simulink model "MatlabNonlinearStateEstimationForActuatorDelay"  (R2020b)
settings: Solver=VariableStepAuto  StartTime=0.0  StopTime=10  RelTol=1e-3
PostLoadFcn:
  | t0 = 0;
values from neighbouring files (symbols this model uses):
  cg = temp(4)    [NonlinearStateEstimationForActuatorDelay.m]
  Croll = Croll_p + .0001 * (rand - 0.5)    [Forces_and_Moments_Calculator.m]
  Cside = 0    [Forces_and_Moments_Calculator.m]
  Cyaw = Cyaw + .1 * (rand - 0.5)    [Forces_and_Moments_Calculator.m]
  F = eye(6)    [MEKFAttitudeOnly.m]
  I = reshape(x(1:9), [3 3])    [AdaptiveLQR.m]    (also in MEKF.m = diag([0.08 0.08 0.002]); MEKFAttitudeOnly.m = diag([0.08 0.08 0.002]); MEKF_old.m = diag([0.08 0.08 0.002]); NonlinearStateEstimationForActuatorDelay.m = diag([Ixx, Ixx, Izz]))
  mass = 1.0565    [ImpactVelocityNotParallelMatlab.m]    (also in NonlinearStateEstimationForActuatorDelay.m = temp(1); OneDLanding.m; RunImpactVelocityParforCompiled.m; Tracker.m = 1.0616753546)
  q = x(13:16)    [AdaptiveLQR.m]    (also in MEKF.m = nominal_state(4:7); MEKFAttitudeOnly.m = [1 0 0 0]; MEKF_old.m = nominal_state(4:7); NonlinearStateEstimationForActuatorDelay.m = x(4:7))
  r = sym('r', [3 1])    [StateSpaceController.m]    (also in TimeDelayCompensationElevator.m = [0;0]; Tracker.m = [0; 0; -(rocket_length - Average_cg)])
  ThrustTable = xlsread('F15_Thrust','Sheet1')    [ImpactVelocityNotParallelMatlab.m]    (also in OneDLanding.m; ParallelImpactVelocity.m; RunImpactVelocityParforCompiled.m)
undefined symbols (not defined in the file or in its folder): Earth, HeightAboveSeaLevel, Light, masscgI, MIL, WGS84
libraries: shared6dof x5, simulink x3, aerolibwind2 x3, vrlib x2, sharedutil x2, aerolibasang x2, shared6dofsys x2, sharedtransform x2, aerolibatmos2 x1, aerolibbdyn x1, aerolibconvert2 x1, aerolibtransform2 x1
(part 1 of 2)
settings Model: SimulationMode=accelerator  Creator=rag  LastModifiedBy=rag
settings OptimizationCC: InitFltsAndDblsToZero=on
settings HardwareCC: ProdLongLongMode=on  TargetLongLongMode=on

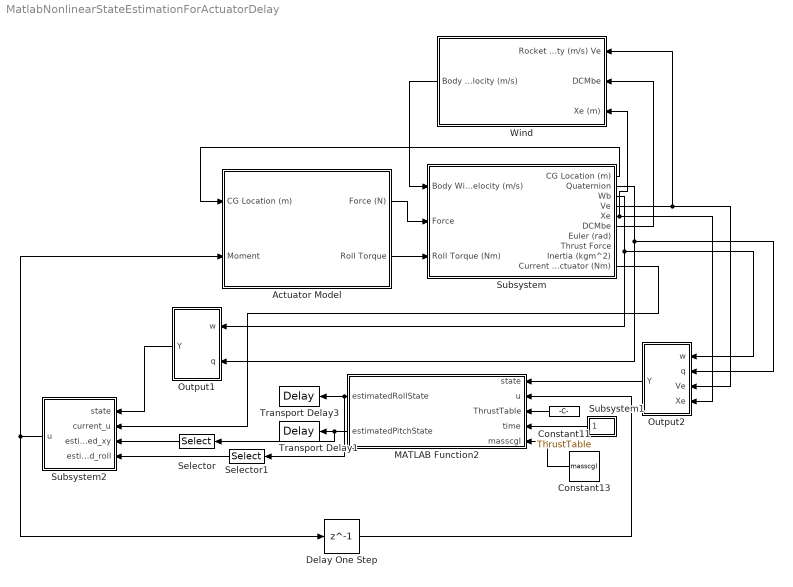
== system MatlabNonlinearStateEstimationForActuatorDelay ==
  Actuator Model : Subsystem
  Constant11 : Constant  Value=ThrustTable
  Constant13 : Constant  Value=masscgI
  Delay One Step : Delay  DelayLength=1
  MATLAB Function2 : MATLAB Function  TreatAsAtomicUnit=on  SystemSampleTime=0.001
  Output1 : Subsystem
  Output2 : Subsystem
  Selector : Selector  InputPortWidth=15  IndexOptions=Index vector (dialog)  Indices=[1:9]  OutputSizes=1
  Selector1 : Selector  InputPortWidth=15  IndexOptions=Index vector (dialog)  Indices=[1:9]  OutputSizes=1
  Subsystem : Subsystem
  Subsystem1 : Subsystem
  Subsystem2 : Subsystem
  Transport Delay1 : TransportDelay  DelayTime=.07  TransDelayFeedthrough=on
  Transport Delay3 : TransportDelay  DelayTime=.01  TransDelayFeedthrough=on
  Wind : Subsystem
  wires:
  Actuator Model/2(Roll Torque) -> Subsystem/3(Roll Torque (Nm))
  Actuator Model/1(Force (N)) -> Subsystem/2(Force)
  Subsystem/1(CG Location (m)) -> Actuator Model/1(CG Location (m))
  Output2/1(Y) -> MATLAB Function2/1(state)
  Subsystem/3(Wb) -> Output2/1(w), Output1/1(w)
  Subsystem/2(Quaternion) -> Output2/2(" q"), Output1/2(" q")
  Subsystem/4(Ve) -> Wind/1(Rocket velocity (m/s) Ve), Output2/3(Ve)
  Subsystem/5(Xe) -> Wind/3(Xe (m)), Output2/4(Xe)
  Subsystem2/1(u) -> Actuator Model/2(Moment), Delay One Step/1
  Constant11/1 -> MATLAB Function2/3(ThrustTable)
  Subsystem1/1(time) -> MATLAB Function2/4(time)
  Constant13/1 -> MATLAB Function2/5(masscgI)
  Output1/1(Y) -> Subsystem2/1(state)
  MATLAB Function2/1(estimatedRollState) -> Transport Delay3/1, Selector1/1
  MATLAB Function2/2(estimatedPitchState) -> Selector/1, Transport Delay1/1
  Delay One Step/1 -> MATLAB Function2/2(u)
  Selector/1 -> Subsystem2/3(estimated_xy)
  Selector1/1 -> Subsystem2/4(estimated_roll)
  Subsystem/10(Current Actuator (Nm)) -> Subsystem2/2(current_u)
  Wind/1(Body Wind Velocity (m/s)) -> Subsystem/1(Body Wind Velocity (m/s))
  Subsystem/6(DCMbe) -> Wind/2(DCMbe)

== system MatlabNonlinearStateEstimationForActuatorDelay/Actuator Model ==
  CG Location (m) : Inport
  Moment : Inport  Port=2
  Constant14 : Constant  Value=[0 1; -1 0]
  Constant3 : Constant  Value=.95
  Demux2 : Demux  Outputs=3
  Force : Product  Multiplication=Matrix(*)
  Moment to Force : Product  Inputs=/*
  Mux2 : Mux  Inputs=2
  Rate Transition : RateTransition  OutPortSampleTime=0.02
  Sum1 : Sum  Inputs=-+|
  Transport Delay : TransportDelay  DelayTime=0.07  TransDelayFeedthrough=on
  Transport Delay1 : TransportDelay  DelayTime=0.01  TransDelayFeedthrough=on
  Force (N) : Outport
  Roll Torque : Outport  Port=2
  wires:
  Demux2/1 -> Mux2/1
  Mux2/1 -> Transport Delay/1
  Sum1/1 -> Moment to Force/1
  Moment to Force/1 -> Force/2
  Constant3/1 -> Sum1/2
  Demux2/2 -> Mux2/2
  Moment/1 -> Demux2/1
  Constant14/1 -> Force/1
  Demux2/3 -> Transport Delay1/1
  CG Location (m)/1 -> Sum1/1
  Force/1 -> Force (N)/1
  Transport Delay/1 -> Moment to Force/2
  Transport Delay1/1 -> Roll Torque/1

== system MatlabNonlinearStateEstimationForActuatorDelay/Output1 ==
  w : Inport
  " q" : Inport  Port=2
  Integrator1 : Integrator
  Selector1 : Selector  InputPortWidth=4  IndexOptions=Index vector (dialog)  Indices=[2 3 4]  OutputSizes=1
  Vector Concatenate4 : Concatenate  NumInputs=3
  Y : Outport  VectorParamsAs1DForOutWhenUnconnected=off
  wires:
  Vector Concatenate4/1 -> Y/1
  w/1 -> Vector Concatenate4/1
  " q"/1 -> Selector1/1
  Integrator1/1 -> Vector Concatenate4/3
  Selector1/1 -> Vector Concatenate4/2, Integrator1/1

== system MatlabNonlinearStateEstimationForActuatorDelay/Output2 ==
  w : Inport
  " q" : Inport  Port=2
  Ve : Inport  Port=3
  Xe : Inport  Port=4
  Integrator1 : Integrator
  Selector1 : Selector  InputPortWidth=4  IndexOptions=Index vector (dialog)  Indices=[2 3 4]  OutputSizes=1
  Vector Concatenate4 : Concatenate  NumInputs=5
  Y : Outport  VectorParamsAs1DForOutWhenUnconnected=off
  wires:
  Vector Concatenate4/1 -> Y/1
  w/1 -> Vector Concatenate4/1
  " q"/1 -> Selector1/1, Vector Concatenate4/2
  Integrator1/1 -> Vector Concatenate4/3
  Selector1/1 -> Integrator1/1
  Xe/1 -> Vector Concatenate4/5
  Ve/1 -> Vector Concatenate4/4

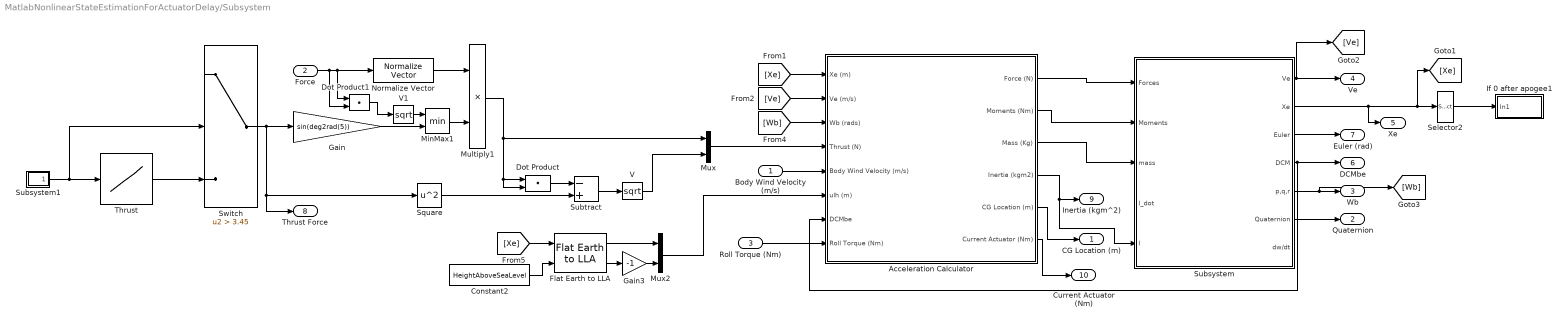
== system MatlabNonlinearStateEstimationForActuatorDelay/Subsystem ==
  Body Wind Velocity (m/s) : Inport
  Force : Inport  Port=2  PortDimensions=2
  Roll Torque (Nm) : Inport  Port=3
  Acceleration Calculator : Subsystem
  Constant2 : Constant  Value=HeightAboveSeaLevel
  Dot Product : DotProduct  SaturateOnIntegerOverflow=on  OutDataTypeStr=Inherit: Inherit via internal rule
  Dot Product1 : DotProduct  SaturateOnIntegerOverflow=on  OutDataTypeStr=Inherit: Inherit via internal rule
  Flat Earth to LLA : aerolibtransform2/Flat Earth to LLA  units=Metric (MKS)  ptype=Earth (WGS84)  F=1/298.257223563  R=6378137  refPosPort=off  LL0=[21.318358277648 -157.9232805920725]  psi=0
  Gain : Gain  Gain=sin(deg2rad(5))
  Gain3 : Gain  Gain=-1
  If 0 after apogee1 : Subsystem
  MinMax1 : MinMax  Inputs=2
  Multiply1 : Product  Inputs=**
  Mux : Mux  Inputs=2
  Mux2 : Mux  Inputs=2
  Normalize Vector : vrlib/Utilities/Normalize Vector  maxzero=0
  Selector2 : Selector  InputPortWidth=3  IndexOptions=Index vector (dialog)  Indices=[3]  OutputSizes=1
  Square : Math  Operator=square  SignedPower=on  SaturateOnIntegerOverflow=on
  Subsystem : Subsystem
  Subsystem1 : Subsystem
  Subtract : Sum  Inputs=-+
  Switch : Switch  Criteria=u2 > Threshold  Threshold=3.45
  Thrust : Lookup_n-D  NumberOfTableDimensions=1  BreakpointsForDimension1=ThrustTable(:,1)  BreakpointsForDimension1FirstPoint=0  BreakpointsForDimension1Spacing=1.5e-5  Table=ThrustTable(:,2)  ExtrapMethod=Clip  InternalRulePriority=Speed  RndMeth=Simplest  InputSameDT=on
  V : Math  Operator=sqrt  SignedPower=on  SaturateOnIntegerOverflow=on
  V1 : Math  Operator=sqrt  SignedPower=on  SaturateOnIntegerOverflow=on
  CG Location (m) : Outport  VectorParamsAs1DForOutWhenUnconnected=off
  Quaternion : Outport  Port=2  VectorParamsAs1DForOutWhenUnconnected=off
  Wb : Outport  Port=3  VectorParamsAs1DForOutWhenUnconnected=off
  Ve : Outport  Port=4  VectorParamsAs1DForOutWhenUnconnected=off
  Xe : Outport  Port=5  VectorParamsAs1DForOutWhenUnconnected=off
  DCMbe : Outport  Port=6  VectorParamsAs1DForOutWhenUnconnected=off
  Euler (rad) : Outport  Port=7  VectorParamsAs1DForOutWhenUnconnected=off
  Thrust Force : Outport  Port=8  VectorParamsAs1DForOutWhenUnconnected=off
  Inertia (kgm^2) : Outport  Port=9  VectorParamsAs1DForOutWhenUnconnected=off
  Current Actuator (Nm) : Outport  Port=10
  wires:
  Flat Earth to LLA/1 -> Mux2/1
  Flat Earth to LLA/2 -> Gain3/1
  Gain3/1 -> Mux2/2
  Mux2/1 -> Acceleration Calculator/6(ulh (m))
  Constant2/1 -> Flat Earth to LLA/2
  [Xe] -> Acceleration Calculator/1(Xe (m))
  Selector2/1 -> If 0 after apogee1/1(In1)
  [Xe] -> Flat Earth to LLA/1
  Acceleration Calculator/5(CG Location (m)) -> CG Location (m)/1
  Acceleration Calculator/4(Inertia (kgm2)) -> Subsystem/5(I), Inertia (kgm^2)/1
  Acceleration Calculator/1(Force (N)) -> Subsystem/1(Forces)
  Roll Torque (Nm)/1 -> Acceleration Calculator/8(Roll Torque (Nm))
  Gain/1 -> MinMax1/2
  Switch/1 -> Thrust Force/1, Square/1, Gain/1
  Subsystem1/1(time) -> Switch/2, Thrust/1
  Subsystem/2(Xe) -> Xe/1, [Xe], Selector2/1
  Subsystem/3(Euler) -> Euler (rad)/1
  Square/1 -> Subtract/2
  Dot Product/1 -> Subtract/1
  V/1 -> Mux/2
  Subtract/1 -> V/1
  Dot Product1/1 -> V1/1
  MinMax1/1 -> Multiply1/2
  Normalize Vector/1 -> Multiply1/1
  V1/1 -> MinMax1/1
  Force/1 -> Dot Product1/2, Dot Product1/1, Normalize Vector/1
  Subsystem/6(Quaternion) -> Quaternion/1
  Subsystem/4(DCM) -> Acceleration Calculator/7(DCMbe), DCMbe/1
  Thrust/1 -> Switch/3
  Acceleration Calculator/2(Moments (Nm)) -> Subsystem/2(Moments)
  Multiply1/1 -> Mux/1, Dot Product/2, Dot Product/1
  Body Wind Velocity (m/s)/1 -> Acceleration Calculator/5(Body Wind Velocity (m/s))
  Acceleration Calculator/3(Mass (Kg)) -> Subsystem/3(mass)
  Subsystem/1(Ve) -> [Ve], Ve/1
  [Ve] -> Acceleration Calculator/2(Ve (m/s))
  Mux/1 -> Acceleration Calculator/4(Thrust (N))
  Subsystem/5(p,q,r) -> [Wb], Wb/1
  [Wb] -> Acceleration Calculator/3(Wb (rads))
  Acceleration Calculator/6(Current Actuator (Nm)) -> Current Actuator (Nm)/1

== system MatlabNonlinearStateEstimationForActuatorDelay/Subsystem1 ==
  Clock : Clock
      settings: Decimation=100
  Constant : Constant  Value=t0
  Sum : Sum  Inputs=|++
  time : Outport
  wires:
  Clock/1 -> Sum/1
  Sum/1 -> time/1
  Constant/1 -> Sum/2

== system MatlabNonlinearStateEstimationForActuatorDelay/Subsystem2 ==
  state : Inport
  current_u : Inport  Port=2
  estimated_xy : Inport  Port=3
  estimated_roll : Inport  Port=4
  Clock : Clock
  MATLAB Function1 : MATLAB Function  TreatAsAtomicUnit=on
  Matrix Multiply : Product  Multiplication=Matrix(*)
  Matrix Multiply1 : Product  Multiplication=Matrix(*)
  Mux : Mux  Inputs=2
  Sum : Sum  Inputs=|--
  u : Outport
  wires:
  Clock/1 -> MATLAB Function1/2(time)
  state/1 -> MATLAB Function1/1(state)
  Sum/1 -> u/1
  MATLAB Function1/3(k_0_out) -> Sum/2
  MATLAB Function1/1(K_x_xy_out) -> Matrix Multiply/1
  current_u/1 -> MATLAB Function1/3(current_u)
  MATLAB Function1/2(K_x_roll_out) -> Matrix Multiply1/1
  estimated_xy/1 -> Matrix Multiply/2
  estimated_roll/1 -> Matrix Multiply1/2
  Matrix Multiply/1 -> Mux/1
  Matrix Multiply1/1 -> Mux/2
  Mux/1 -> Sum/1

== system MatlabNonlinearStateEstimationForActuatorDelay/Wind ==
  Rocket velocity (m/s) Ve : Inport
  DCMbe : Inport  Port=2
  Xe (m) : Inport  Port=3
  Constant : Constant  Commented=on  Value=2
  Ground : Ground  Commented=on
  Mux : Mux  Commented=on  Inputs=3
  Sel2 : Selector  InputPortWidth=3  IndexOptions=Index vector (dialog)  Indices=3  OutputSizes=1
  Subsystem3 : Subsystem
  Terminator : Terminator
  transform to body axes : shared6dof/6DOF (Euler Angles)/transform to Inertial axes   Commented=on  SystemSampleTime=-1  VariantActivationTime=update diagram  Latency=0  AutoFrameSizeCalculation=off
      settings: SourceProductBaseCode=AE,PW,MT,UV,VE,VP
  Body Wind Velocity (m/s) : Outport  VectorParamsAs1DForOutWhenUnconnected=off
  wires:
  DCMbe/1 -> Subsystem3/3(DCMbe), transform to body axes/2
  Rocket velocity (m/s) Ve/1 -> Subsystem3/1(Rocket velocity (m/s) Ve)
  Mux/1 -> transform to body axes/1
  Xe (m)/1 -> Sel2/1
  Constant/1 -> Mux/1
  Subsystem3/1(wind angular velocity (rad/s)) -> Terminator/1
  Sel2/1 -> Subsystem3/2(height (m))
  Ground/1 -> Mux/2, Mux/3
  Subsystem3/2(body axis wind velocity (m/s)) -> Body Wind Velocity (m/s)/1

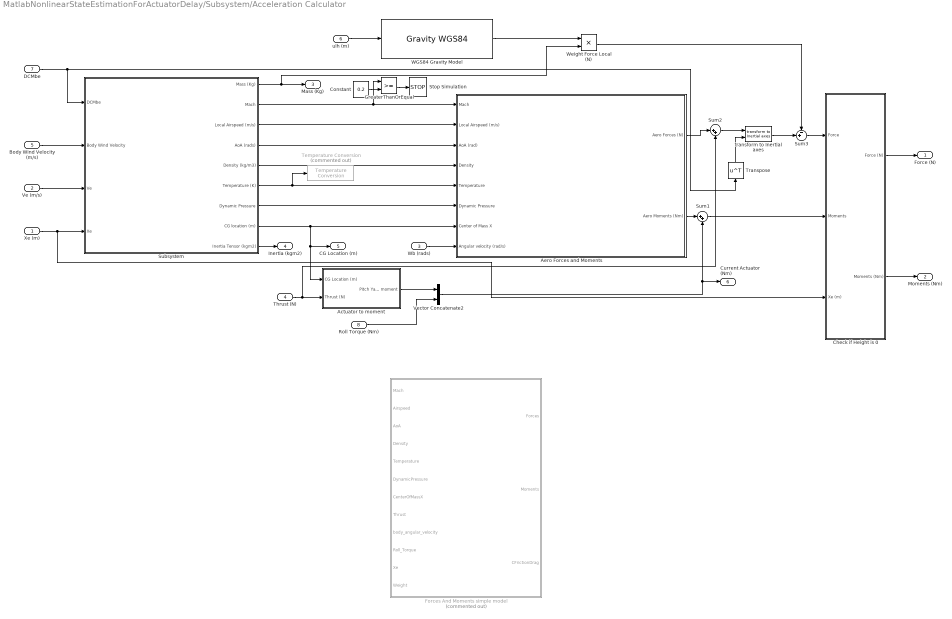
== system MatlabNonlinearStateEstimationForActuatorDelay/Subsystem/Acceleration Calculator ==
  Xe (m) : Inport
  Ve (m/s) : Inport  Port=2
  Wb (rads) : Inport  Port=3
  Thrust (N) : Inport  Port=4
  Body Wind Velocity (m/s) : Inport  Port=5
  ulh (m) : Inport  Port=6  PortDimensions=3
  DCMbe : Inport  Port=7
  Roll Torque (Nm) : Inport  Port=8
  Actuator to moment : Subsystem
  Aero Forces and Moments : Subsystem
  Check if Height is 0 : Subsystem
  Constant : Constant  Value=0.2
  Forces And Moments simple model : MATLAB Function  Commented=on  TreatAsAtomicUnit=on
  GreaterThanOrEqual : RelationalOperator  OutDataTypeStr=boolean  RndMeth=Simplest
  Stop Simulation : Stop
  Subsystem : Subsystem
  Sum1 : Sum  Inputs=|++
  Sum2 : Sum  Inputs=|++
  Sum3 : Sum  Inputs=-+|
  Temperature Conversion : aerolibconvert2/Temperature Conversion  Commented=on  IU=K  OU=C
      settings: SourceProductBaseCode=AE
  Transpose : Math  Operator=transpose  SignedPower=on  SaturateOnIntegerOverflow=on
  Vector Concatenate2 : Concatenate
  "WGS84 Gravity Model  " : GravityWGS84
  Weight Force Local (N) : Product
  "transform to Inertial axes " : shared6dof/6DOF (Euler Angles)/transform to Inertial axes   SystemSampleTime=-1  VariantActivationTime=update diagram  Latency=0  AutoFrameSizeCalculation=off
      settings: SourceProductBaseCode=AE,PW,MT,UV,VE,VP
  Force (N) : Outport  VectorParamsAs1DForOutWhenUnconnected=off
  Moments (Nm) : Outport  Port=2  VectorParamsAs1DForOutWhenUnconnected=off
  Mass (Kg) : Outport  Port=3  VectorParamsAs1DForOutWhenUnconnected=off
  Inertia (kgm2) : Outport  Port=4  VectorParamsAs1DForOutWhenUnconnected=off
  CG Location (m) : Outport  Port=5  VectorParamsAs1DForOutWhenUnconnected=off
  Current Actuator (Nm) : Outport  Port=6
  wires:
  Ve (m/s)/1 -> Subsystem/3(Ve)
  Subsystem/9(Inertia Tensor (kgm2)) -> Inertia (kgm2)/1
  Subsystem/1(Mass (Kg)) -> Weight Force Local (N)/2, Mass (Kg)/1
  DCMbe/1 -> Transpose/1, Subsystem/1(DCMbe)
  ulh (m)/1 -> "WGS84 Gravity Model  "/1
  Roll Torque (Nm)/1 -> Vector Concatenate2/2
  Thrust (N)/1 -> Sum2/2, Actuator to moment/2(Thrust (N))
  Actuator to moment/1(Pitch Yaw moment) -> Vector Concatenate2/1
  Xe (m)/1 -> Subsystem/4(Xe), Check if Height is 0/3(Xe (m))
  Subsystem/3(Local Airspeed (m/s)) -> Aero Forces and Moments/2(Local Airspeed (m/s))
  Subsystem/2(Mach) -> GreaterThanOrEqual/1, Aero Forces and Moments/1(Mach)
  Subsystem/4(AoA (rads)) -> Aero Forces and Moments/3(AoA (rad))
  Subsystem/5(Density (kg/m3)) -> Aero Forces and Moments/4(Density)
  Subsystem/6(Temperature (K)) -> Temperature Conversion/1, Aero Forces and Moments/5(Temperature)
  Subsystem/7(Dynamic Pressure) -> Aero Forces and Moments/6(Dynamic Pressure)
  Subsystem/8(CG location (m)) -> Aero Forces and Moments/7(Center of Mass X), Actuator to moment/1(CG Location (m)), CG Location (m)/1
  Wb (rads)/1 -> Aero Forces and Moments/8(Angular velocity (rad/s))
  Aero Forces and Moments/1(Aero Forces (N)) -> Sum2/1
  Weight Force Local (N)/1 -> Sum3/1
  Sum1/1 -> Check if Height is 0/2(Moments)
  Sum2/1 -> "transform to Inertial axes "/1
  Check if Height is 0/1(Force (N)) -> Force (N)/1
  Check if Height is 0/2(Moments (Nm)) -> Moments (Nm)/1
  Body Wind Velocity (m/s)/1 -> Subsystem/2(Body Wind Velocity)
  "WGS84 Gravity Model  "/1 -> Weight Force Local (N)/1
  Constant/1 -> GreaterThanOrEqual/2
  GreaterThanOrEqual/1 -> Stop Simulation/1
  Transpose/1 -> "transform to Inertial axes "/2
  "transform to Inertial axes "/1 -> Sum3/2
  Sum3/1 -> Check if Height is 0/1(Force)
  Aero Forces and Moments/2(Aero Moments (Nm)) -> Sum1/1
  Vector Concatenate2/1 -> Current Actuator (Nm)/1, Sum1/2

== system MatlabNonlinearStateEstimationForActuatorDelay/Subsystem/If 0 after apogee1 ==
  In1 : Inport
  Compare To Zero1 : simulink/Logic and Bit Operations/Compare To Zero  relop=<=  OutDataTypeStr=boolean
  Constant3 : Constant  Value=0.5
  Logical Operator1 : Logic  AllPortsSameDT=off  OutDataTypeStr=boolean
  Relational Operator1 : RelationalOperator  Operator=>  OutDataTypeStr=boolean  RndMeth=Simplest
  Stop Simulation1 : Stop
  Subsystem1 : Subsystem
  wires:
  Constant3/1 -> Relational Operator1/2
  In1/1 -> Compare To Zero1/1
  Logical Operator1/1 -> Stop Simulation1/1
  Compare To Zero1/1 -> Logical Operator1/2
  Relational Operator1/1 -> Logical Operator1/1
  Subsystem1/1(time) -> Relational Operator1/1

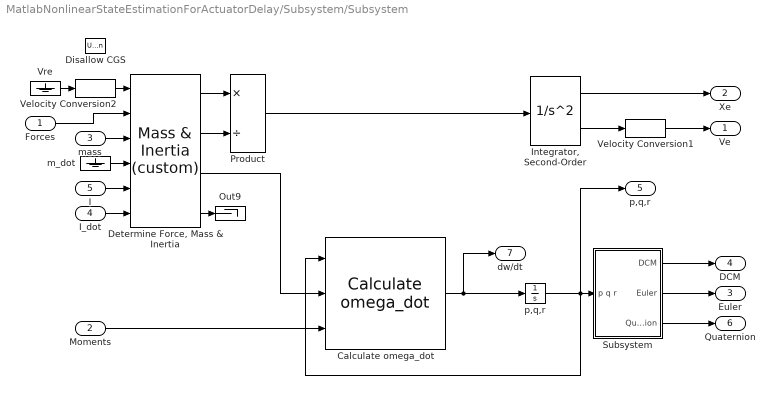
== system MatlabNonlinearStateEstimationForActuatorDelay/Subsystem/Subsystem ==
  Forces : Inport  Unit=N  PortDimensions=3
  Moments : Inport  Port=2  Unit=N*m  PortDimensions=3
  mass : Inport  Port=3  Unit=kg
  I_dot : Inport  Port=4  Unit=kg*m^2/s  PortDimensions=[3 3]
  I : Inport  Port=5  Unit=kg*m^2  PortDimensions=[3 3]
  Calculate omega_dot : shared6dofsys/Calculate omega_dot  aMode=aMode
      settings: SourceProductBaseCode=AE,PW,MT,UV,VE,VP
  "Determine Force, Mass & Inertia" : shared6dofsys/Mass & Inertia (custom)  aMode=aMode
      settings: SourceProductBaseCode=AE,PW,MT,UV,VE,VP
  Disallow CGS : UnitConfiguration  UnitSystemsStr=English,SI,SI (extended)  AllowAllUnitSystems=off
  "Integrator, Second-Order" : SecondOrderIntegrator  ICX=[0 0 50]  LimitX=on  LowerLimitX=[-inf -inf 0]  ICDXDT=0
  Out9 : Terminator
  Product : Product  Inputs=*/  SaturateOnIntegerOverflow=on  OutDataTypeStr=Inherit: Same as first input
  Subsystem : Subsystem
  Velocity Conversion1 : shared6dof/6DOF (Euler Angles)/Velocity Conversion1  SystemSampleTime=-1  VariantActivationTime=update diagram  Latency=0  AutoFrameSizeCalculation=off
      settings: SourceProductBaseCode=AE,PW,MT,UV,VE,VP
  Velocity Conversion2 : shared6dof/6DOF (Euler Angles)/Velocity Conversion2  SystemSampleTime=-1  VariantActivationTime=update diagram  Latency=0  AutoFrameSizeCalculation=off
      settings: SourceProductBaseCode=AE,PW,MT,UV,VE,VP
  Vre : Ground
  m_dot : Ground
  "p,q,r " : Integrator  InitialCondition=[0 0 0]
  Ve : Outport  Unit=m/s  VectorParamsAs1DForOutWhenUnconnected=off
  Xe : Outport  Port=2  Unit=m  VectorParamsAs1DForOutWhenUnconnected=off
  Euler : Outport  Port=3  Unit=rad  VectorParamsAs1DForOutWhenUnconnected=off
  DCM : Outport  Port=4  Unit=1  VectorParamsAs1DForOutWhenUnconnected=off
  p,q,r : Outport  Port=5  Unit=rad/s  VectorParamsAs1DForOutWhenUnconnected=off
  Quaternion : Outport  Port=6  VectorParamsAs1DForOutWhenUnconnected=off
  dw/dt : Outport  Port=7  VectorParamsAs1DForOutWhenUnconnected=off
  wires:
  Subsystem/2(Euler) -> Euler/1
  "Determine Force, Mass & Inertia"/3 -> Calculate omega_dot/2
  "p,q,r "/1 -> Subsystem/1(p q r), p,q,r/1, Calculate omega_dot/1
  Product/1 -> "Integrator, Second-Order"/1
  mass/1 -> "Determine Force, Mass & Inertia"/3
  Velocity Conversion1/1 -> Ve/1
  Subsystem/1(DCM) -> DCM/1
  Calculate omega_dot/1 -> dw/dt/1, "p,q,r "/1
  Forces/1 -> "Determine Force, Mass & Inertia"/2
  "Determine Force, Mass & Inertia"/4 -> Out9/1
  I_dot/1 -> "Determine Force, Mass & Inertia"/6
  I/1 -> "Determine Force, Mass & Inertia"/5
  Velocity Conversion2/1 -> "Determine Force, Mass & Inertia"/1
  Vre/1 -> Velocity Conversion2/1
  "Determine Force, Mass & Inertia"/1 -> Product/1
  "Determine Force, Mass & Inertia"/2 -> Product/2
  m_dot/1 -> "Determine Force, Mass & Inertia"/4
  Subsystem/3(Quaternion) -> Quaternion/1
  "Integrator, Second-Order"/2 -> Velocity Conversion1/1
  "Integrator, Second-Order"/1 -> Xe/1
  Moments/1 -> Calculate omega_dot/3

== system MatlabNonlinearStateEstimationForActuatorDelay/Subsystem/Subsystem1 ==
  Clock : Clock
      settings: Decimation=100
  Constant : Constant  Value=t0
  Sum : Sum  Inputs=|++
  time : Outport
  wires:
  Clock/1 -> Sum/1
  Sum/1 -> time/1
  Constant/1 -> Sum/2

== system MatlabNonlinearStateEstimationForActuatorDelay/Wind/Subsystem3 ==
  Rocket velocity (m/s) Ve : Inport
  height (m) : Inport  Port=2
  DCMbe : Inport  Port=3
  Discrete Wind Gust Model : aerolibwind2/Discrete Wind Gust Model  units=Metric (MKS)  Gx=on  Gy=on  Gz=on  t_0=GustStart  d_m=GustLength  v_m=GuestAmplitude
  Dot Product : DotProduct  SaturateOnIntegerOverflow=on  OutDataTypeStr=Inherit: Inherit via internal rule
  Sum : Sum  Inputs=3
  V : Math  Operator=sqrt  SignedPower=on  SaturateOnIntegerOverflow=on
  Von Karman Wind Turbulence Model (Continuous (+q +r)) : aerolibwind2/Dryden Wind Turbulence Model  (Continuous (+q -r))  units=Metric (MKS)  spec=MIL-F-8785C  model=Discrete Dryden (+q -r)  W20=ShearSpeed  Wdeg=ShearDirection  TurbProb=10^-2 - Light  L_high=762  Wingspan=1  ts=0.1  Seed=[23341 23342 23343 23344]  T_on=on
  Wind Shear Model : aerolibwind2/Wind Shear Model  units=Metric (MKS)  phase=Category C - Terminal Flight Phase  W_20=ShearSpeed  Wdeg=ShearDirection
  wind angular velocity (rad/s) : Outport  VectorParamsAs1DForOutWhenUnconnected=off
  body axis wind velocity (m/s) : Outport  Port=2  VectorParamsAs1DForOutWhenUnconnected=off
  wires:
  height (m)/1 -> Wind Shear Model/1, Von Karman Wind Turbulence Model (Continuous (+q +r))/1
  Discrete Wind Gust Model/1 -> Sum/1
  DCMbe/1 -> Wind Shear Model/2, Von Karman Wind Turbulence Model (Continuous (+q +r))/3
  V/1 -> Von Karman Wind Turbulence Model (Continuous (+q +r))/2, Discrete Wind Gust Model/1
  Sum/1 -> body axis wind velocity (m/s)/1
  Wind Shear Model/1 -> Sum/3
  Von Karman Wind Turbulence Model (Continuous (+q +r))/1 -> Sum/2
  Von Karman Wind Turbulence Model (Continuous (+q +r))/2 -> wind angular velocity (rad/s)/1
  Dot Product/1 -> V/1
  Rocket velocity (m/s) Ve/1 -> Dot Product/1, Dot Product/2

== system MatlabNonlinearStateEstimationForActuatorDelay/Subsystem/Acceleration Calculator/Actuator to moment ==
  CG Location (m) : Inport
  Thrust (N) : Inport  Port=2
  1 : Constant  Value=[0 0]
  Constant : Constant  Value=0
  Constant3 : Constant  Value=.95
  Cross Product : vrlib/Utilities/Cross Product
  Get Actuator Force : Selector  InputPortWidth=3  IndexOptions=Index vector (dialog)  Indices=[1 2]  OutputSizes=1
  Get Actuator Force1 : Selector  InputPortWidth=3  IndexOptions=Index vector (dialog)  Indices=[1 2]  OutputSizes=1
  Mux : Mux  Inputs=2
  Mux1 : Mux  Inputs=2
  Sum1 : Sum  Inputs=-+|
  Pitch Yaw moment : Outport  VectorParamsAs1DForOutWhenUnconnected=off
  wires:
  Constant3/1 -> Sum1/2
  Get Actuator Force/1 -> Mux1/1
  CG Location (m)/1 -> Sum1/1
  Thrust (N)/1 -> Get Actuator Force/1
  Cross Product/1 -> Get Actuator Force1/1
  Mux/1 -> Cross Product/1
  Sum1/1 -> Mux/2
  1/1 -> Mux/1
  Mux1/1 -> Cross Product/2
  Constant/1 -> Mux1/2
  Get Actuator Force1/1 -> Pitch Yaw moment/1

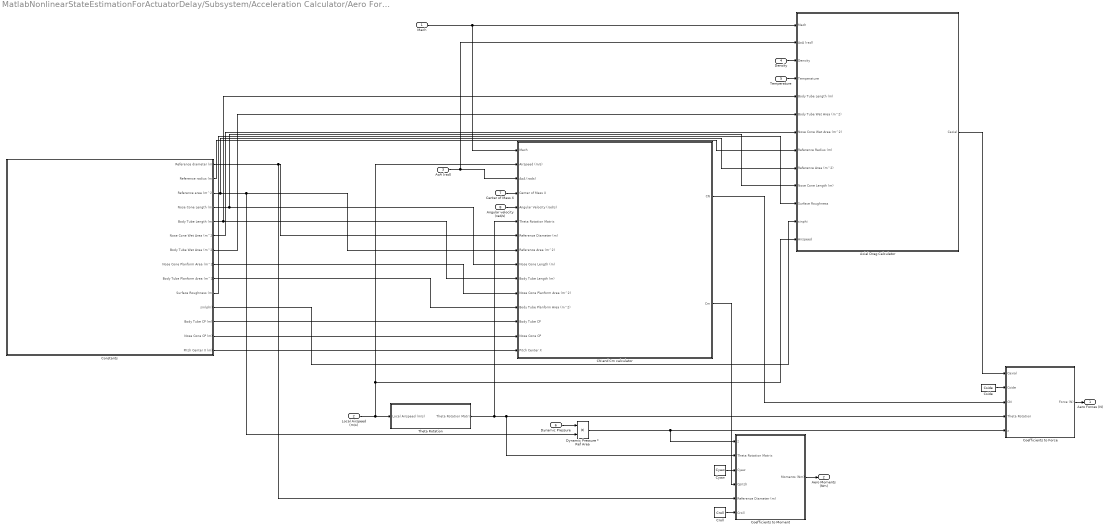
== system MatlabNonlinearStateEstimationForActuatorDelay/Subsystem/Acceleration Calculator/Aero Forces and Moments ==
  Mach : Inport
  Local Airspeed (m/s) : Inport  Port=2
  AoA (rad) : Inport  Port=3
  Density : Inport  Port=4
  Temperature : Inport  Port=5
  Dynamic Pressure : Inport  Port=6
  Center of Mass X : Inport  Port=7
  Angular velocity (rad/s) : Inport  Port=8
  Axial Drag Calculator : Subsystem
  CN and Cm calculator : Subsystem
  Coefficients to Force : Subsystem
  Coefficients to Moment : Subsystem
  Constants : Subsystem
  Croll : Constant  Value=Croll
  Cside : Constant  Value=Cside
  Cyaw : Constant  Value=Cyaw
  Dynamic Pressure * Ref Area : Product
  Theta Rotation : Subsystem
  Aero Forces (N) : Outport  VectorParamsAs1DForOutWhenUnconnected=off
  Aero Moments (Nm) : Outport  Port=2  VectorParamsAs1DForOutWhenUnconnected=off
  wires:
  AoA (rad)/1 -> Axial Drag Calculator/2(AoA (rad)), CN and Cm calculator/3(AoA (rads))
  Temperature/1 -> Axial Drag Calculator/4(Temperature)
  Coefficients to Force/1(Force (N)) -> Aero Forces (N)/1
  Mach/1 -> Axial Drag Calculator/1(Mach), CN and Cm calculator/1(Mach)
  CN and Cm calculator/1(CN) -> Coefficients to Force/3(CN)
  Angular velocity (rad/s)/1 -> CN and Cm calculator/5(Angular Velocity (rad/s))
  Center of Mass X/1 -> CN and Cm calculator/4(Center of Mass X)
  Axial Drag Calculator/1(Caxial) -> Coefficients to Force/1(Caxial)
  Dynamic Pressure/1 -> Dynamic Pressure * Ref Area/1
  Local Airspeed (m/s)/1 -> Axial Drag Calculator/13(Airspeed), CN and Cm calculator/2(Airspeed (m/s)), Theta Rotation/1(Local Airspeed (m/s))
  Cside/1 -> Coefficients to Force/2(Cside)
  Coefficients to Moment/1(Moments (Nm)) -> Aero Moments (Nm)/1
  CN and Cm calculator/2(Cm) -> Coefficients to Moment/4(Cpitch)
  Theta Rotation/1(Theta Rotation Matrix) -> Coefficients to Moment/2(Theta Rotation Matrix), Coefficients to Force/4(Theta Rotation), CN and Cm calculator/6(Theta Rotation Matrix)
  Dynamic Pressure * Ref Area/1 -> Coefficients to Force/5(z), Coefficients to Moment/1(z)
  Constants/1(Reference diameter (m)) -> CN and Cm calculator/7(Reference Diameter (m)), Coefficients to Moment/5(Reference Diameter (m))
  Constants/3(Reference area (m^2)) -> Dynamic Pressure * Ref Area/2, CN and Cm calculator/8(Reference Area (m^2)), Axial Drag Calculator/9(Reference Area (m^2))
  Constants/4(Nose Cone Length (m)) -> Axial Drag Calculator/10(Nose Cone Length (m)), CN and Cm calculator/9(Nose Cone Length (m))
  Constants/5(Body Tube Length (m)) -> Axial Drag Calculator/5(Body Tube Length (m)), CN and Cm calculator/10(Body Tube Length (m))
  Constants/8(Nose Cone Planform Area (m^2)) -> CN and Cm calculator/11(Nose Cone Planform Area (m^2))
  Constants/9(Body Tube Planform Area (m^2)) -> CN and Cm calculator/12(Body Tube Planform Area (m^2))
  Constants/12(Body Tube CP (m)) -> CN and Cm calculator/13(Body Tube CP)
  Constants/13(Nose Cone CP (m)) -> CN and Cm calculator/14(Nose Cone CP)
  Constants/14(Pitch Center X (m)) -> CN and Cm calculator/15(Pitch Center X)
  Constants/7(Body Tube Wet Area (m^2)) -> Axial Drag Calculator/6(Body Tube Wet Area (m^2))
  Constants/6("Nose Cone Wet Area (m^2) ") -> Axial Drag Calculator/7(Nose Cone Wet Area (m^2))
  Constants/2(Reference radius (m)) -> Axial Drag Calculator/8(Reference Radius (m))
  Constants/10(Surface Roughness (m)) -> Axial Drag Calculator/11(Surface Roughness)
  Constants/11(sin(phi)) -> Axial Drag Calculator/12(sinphi)
  Density/1 -> Axial Drag Calculator/3(Density)
  Cyaw/1 -> Coefficients to Moment/3(Cyaw)
  Croll/1 -> Coefficients to Moment/6(Croll)

== system MatlabNonlinearStateEstimationForActuatorDelay/Subsystem/Acceleration Calculator/Check if Height is 0 ==
  Force : Inport
  Moments : Inport  Port=2
  Xe (m) : Inport  Port=3
  0,3 : Constant  Value=[0;0;0]
  1 : Constant  Value=[0 0]
  2 : Constant  Value=0
  Height : Selector  InputPortWidth=3  IndexOptions=Index vector (dialog)  Indices=3  OutputSizes=1
  If on ground : Switch  Criteria=u2 > Threshold
  If on ground and force is not up : Switch  Criteria=u2 > Threshold
  Mux : Mux  Inputs=2
  Selector : Selector  InputPortWidth=3  IndexOptions=Index vector (dialog)  Indices=3  OutputSizes=1
  mul3 : Switch  Criteria=u2 ~= 0  Threshold=deg2rad(17)
  Force (N) : Outport  VectorParamsAs1DForOutWhenUnconnected=off
  Moments (Nm) : Outport  Port=2  VectorParamsAs1DForOutWhenUnconnected=off
  wires:
  Moments/1 -> mul3/1
  Force/1 -> If on ground/1, Selector/1
  Xe (m)/1 -> Height/1
  0,3/1 -> mul3/3
  Height/1 -> If on ground/2, mul3/2
  2/1 -> If on ground and force is not up/3
  Selector/1 -> If on ground and force is not up/1, If on ground and force is not up/2
  1/1 -> Mux/1
  Mux/1 -> If on ground/3
  If on ground and force is not up/1 -> Mux/2
  If on ground/1 -> Force (N)/1
  mul3/1 -> Moments (Nm)/1

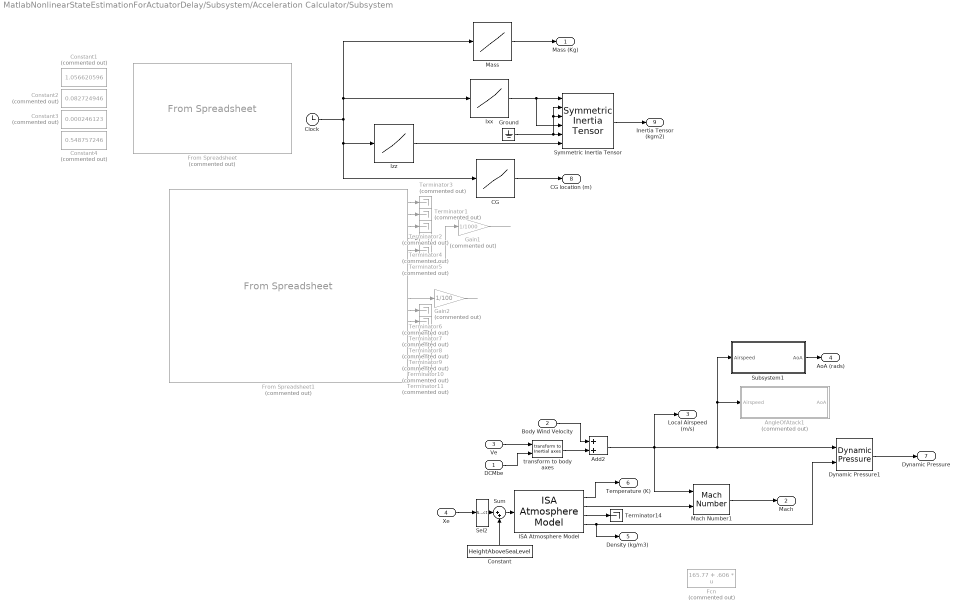
== system MatlabNonlinearStateEstimationForActuatorDelay/Subsystem/Acceleration Calculator/Subsystem ==
  DCMbe : Inport
  Body Wind Velocity : Inport  Port=2
  Ve : Inport  Port=3
  Xe : Inport  Port=4
  Add2 : Sum
  AngleOfAtack1 : MATLAB Function  Commented=on  TreatAsAtomicUnit=on
  CG : Lookup_n-D  NumberOfTableDimensions=1  BreakpointsForDimension1=masscgI(:,1)  BreakpointsForDimension1FirstPoint=0  BreakpointsForDimension1Spacing=1.5e-5  Table=masscgI(:,5)  ExtrapMethod=Clip  InternalRulePriority=Speed  RndMeth=Simplest  InputSameDT=on
  Clock : Clock
  Constant : Constant  Value=HeightAboveSeaLevel
  Constant1 : Constant  Commented=on  Value=1.056620596
  Constant2 : Constant  Commented=on  Value=0.082724946
  Constant3 : Constant  Commented=on  Value=0.000246123
  Constant4 : Constant  Commented=on  Value=0.548757246
  Dynamic Pressure1 : aerolibasang/Dynamic Pressure
  Fcn : Fcn  Commented=on  Expr=165.77 + .606 * u
  From Spreadsheet : FromSpreadsheet  Commented=on  FileName=mass,cg,I.xlsx  SheetName=mass,cg,I  Range=A1:E4395  ExtrapolationBeforeFirstDataPoint=Hold first value  InterpolationWithinTimeRange=Zero order hold  ExtrapolationAfterLastDataPoint=Hold last value
  From Spreadsheet1 : FromSpreadsheet  Commented=on  FileName=cg mass MOI.xlsx  SheetName=cg mass MOI  Range=A1:E4395  ExtrapolationBeforeFirstDataPoint=Hold first value  ExtrapolationAfterLastDataPoint=Hold last value
  Gain1 : Gain  Commented=on  Gain=1/1000
  Gain2 : Gain  Commented=on  Gain=1/100
  Ground : Ground
  ISA Atmosphere Model : aerolibatmos2/ISA Atmosphere Model  custom=on  g=9.80665  gamma=1.4  R=287.0531  L=0.0065  h_trop=11000  h_strat=20000  rho0=1.225  P0=101325  T0=288.15  h0=0
  Ixx : Lookup_n-D  NumberOfTableDimensions=1  BreakpointsForDimension1=masscgI(:,1)  BreakpointsForDimension1FirstPoint=0  BreakpointsForDimension1Spacing=1.5e-5  Table=masscgI(:,3)  ExtrapMethod=Clip  InternalRulePriority=Speed  RndMeth=Simplest  InputSameDT=on
  Izz : Lookup_n-D  NumberOfTableDimensions=1  BreakpointsForDimension1=masscgI(:,1)  BreakpointsForDimension1FirstPoint=0  BreakpointsForDimension1Spacing=1.5e-5  Table=masscgI(:,4)  ExtrapMethod=Clip  InternalRulePriority=Speed  RndMeth=Simplest  InputSameDT=on
  Mach Number1 : aerolibasang/Mach Number
      settings: SourceProductBaseCode=AE
  Mass : Lookup_n-D  NumberOfTableDimensions=1  BreakpointsForDimension1=masscgI(:,1)  BreakpointsForDimension1FirstPoint=0  BreakpointsForDimension1Spacing=1.5e-5  Table=masscgI(:,2)  ExtrapMethod=Clip  InternalRulePriority=Speed  RndMeth=Simplest  InputSameDT=on
  Sel2 : Selector  InputPortWidth=3  IndexOptions=Index vector (dialog)  Indices=3  OutputSizes=1
  Subsystem1 : Subsystem
  Sum : Sum  Inputs=|++
  Symmetric Inertia Tensor : aerolibbdyn/Symmetric Inertia Tensor
      settings: SourceProductBaseCode=AE
  Terminator{1..11} (11 alike) : Terminator  Commented=on
  Terminator14 : Terminator
  "transform to body axes " : shared6dof/6DOF (Euler Angles)/transform to Inertial axes   SystemSampleTime=-1  VariantActivationTime=update diagram  Latency=0  AutoFrameSizeCalculation=off
      settings: SourceProductBaseCode=AE,PW,MT,UV,VE,VP
  Mass (Kg) : Outport  VectorParamsAs1DForOutWhenUnconnected=off
  Mach : Outport  Port=2  VectorParamsAs1DForOutWhenUnconnected=off
  Local Airspeed (m/s) : Outport  Port=3  VectorParamsAs1DForOutWhenUnconnected=off
  AoA (rads) : Outport  Port=4  VectorParamsAs1DForOutWhenUnconnected=off
  Density (kg/m3) : Outport  Port=5  VectorParamsAs1DForOutWhenUnconnected=off
  Temperature (K) : Outport  Port=6  VectorParamsAs1DForOutWhenUnconnected=off
  Dynamic Pressure : Outport  Port=7  VectorParamsAs1DForOutWhenUnconnected=off
  CG location (m) : Outport  Port=8  VectorParamsAs1DForOutWhenUnconnected=off
  Inertia Tensor (kgm2) : Outport  Port=9  VectorParamsAs1DForOutWhenUnconnected=off
  wires:
  From Spreadsheet1/4 -> Terminator4/1
  ISA Atmosphere Model/4 -> Density (kg/m3)/1, Dynamic Pressure1/2
  From Spreadsheet1/5 -> Terminator5/1
  From Spreadsheet1/9 -> Gain2/1
  From Spreadsheet1/6 -> Gain1/1
  Dynamic Pressure1/1 -> Dynamic Pressure/1
  Mach Number1/1 -> Mach/1
  From Spreadsheet1/12 -> Terminator8/1
  ISA Atmosphere Model/3 -> Terminator14/1
  Gain2/1 -> ?
  From Spreadsheet1/11 -> Terminator7/1
  Xe/1 -> Sel2/1
  From Spreadsheet1/3 -> Terminator2/1
  From Spreadsheet1/14 -> Terminator10/1
  From Spreadsheet1/2 -> Terminator1/1
  From Spreadsheet1/1 -> Terminator3/1
  From Spreadsheet1/13 -> Terminator9/1
  From Spreadsheet1/15 -> Terminator11/1
  Gain1/1 -> ?
  Ground/1 -> Symmetric Inertia Tensor/2, Symmetric Inertia Tensor/3, Symmetric Inertia Tensor/5
  Symmetric Inertia Tensor/1 -> Inertia Tensor (kgm2)/1
  From Spreadsheet1/10 -> Terminator6/1
  Sel2/1 -> Sum/1
  Ve/1 -> "transform to body axes "/1
  DCMbe/1 -> "transform to body axes "/2
  Add2/1 -> Local Airspeed (m/s)/1, Subsystem1/1(Airspeed), AngleOfAtack1/1(Airspeed), Dynamic Pressure1/1, Mach Number1/1
  Subsystem1/1(AoA) -> AoA (rads)/1
  "transform to body axes "/1 -> Add2/2
  Clock/1 -> Izz/1, CG/1, Ixx/1, Mass/1
  Body Wind Velocity/1 -> Add2/1
  ISA Atmosphere Model/1 -> Temperature (K)/1
  ISA Atmosphere Model/2 -> Mach Number1/2
  Mass/1 -> Mass (Kg)/1
  Ixx/1 -> Symmetric Inertia Tensor/4, Symmetric Inertia Tensor/1
  Izz/1 -> Symmetric Inertia Tensor/6
  CG/1 -> CG location (m)/1
  Sum/1 -> ISA Atmosphere Model/1
  Constant/1 -> Sum/2

== system MatlabNonlinearStateEstimationForActuatorDelay/Subsystem/If 0 after apogee1/Subsystem1 ==
  Clock : Clock
      settings: Decimation=100
  Constant : Constant  Value=t0
  Sum : Sum  Inputs=|++
  time : Outport
  wires:
  Clock/1 -> Sum/1
  Sum/1 -> time/1
  Constant/1 -> Sum/2

== system MatlabNonlinearStateEstimationForActuatorDelay/Subsystem/Subsystem/Subsystem ==
  p q r : Inport
  Quaternion Normalize : sharedutil/Quaternion Normalize  aMode=aMode
      settings: SourceProductBaseCode=AE,PW,MT,UV,VE,VP
  Quaternions to Direction Cosine Matrix : sharedtransform/Quaternions to  Direction Cosine Matrix  aMode=aMode
      settings: SourceProductBaseCode=AE,PW,MT,UV,VE,VP
  Quaternions to Rotation Angles : sharedtransform/Quaternions to Rotation Angles  rotationOrder=ZYX  aMode=aMode
      settings: SourceProductBaseCode=AE,PW,MT,UV,VE,VP
  Selector : Selector  IndexMode=Zero-based  InputPortWidth=3  IndexOptions=Index vector (dialog)  Indices=[ 2 1 0]  OutputSizes=1
  Subsystem : Subsystem
  q0 q1 q2 q3 : Integrator  InitialCondition=[.9 0.2 0 0.5]
  DCM : Outport  VectorParamsAs1DForOutWhenUnconnected=off
  Euler : Outport  Port=2  VectorParamsAs1DForOutWhenUnconnected=off
  Quaternion : Outport  Port=3  VectorParamsAs1DForOutWhenUnconnected=off
  wires:
  Selector/1 -> Euler/1
  q0 q1 q2 q3/1 -> Quaternion Normalize/1
  Quaternions to Direction Cosine Matrix/1 -> DCM/1
  Subsystem/1(qdot1) -> q0 q1 q2 q3/1
  p q r/1 -> Subsystem/1(p q r1)
  Quaternions to Rotation Angles/1 -> Selector/1
  Quaternion Normalize/1 -> Quaternion/1, Subsystem/2(q0 q1 q2 q1), Quaternions to Rotation Angles/1, Quaternions to Direction Cosine Matrix/1

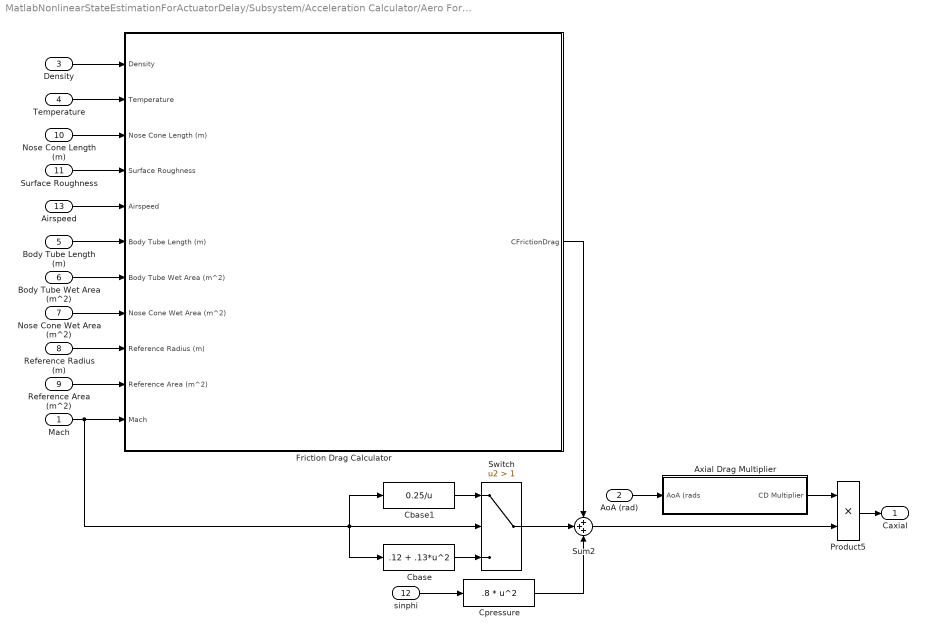
== system MatlabNonlinearStateEstimationForActuatorDelay/Subsystem/Acceleration Calculator/Aero Forces and Moments/Axial Drag Calculator ==
  Mach : Inport
  AoA (rad) : Inport  Port=2
  Density : Inport  Port=3
  Temperature : Inport  Port=4
  Body Tube Length (m) : Inport  Port=5
  Body Tube Wet Area (m^2) : Inport  Port=6
  Nose Cone Wet Area (m^2) : Inport  Port=7
  Reference Radius (m) : Inport  Port=8
  Reference Area (m^2) : Inport  Port=9
  Nose Cone Length (m) : Inport  Port=10
  Surface Roughness : Inport  Port=11
  sinphi : Inport  Port=12
  Airspeed : Inport  Port=13
  Axial Drag Multiplier : Subsystem
  Cbase : Fcn  Expr=.12 + .13*u^2
  Cbase1 : Fcn  Expr=0.25/u
  Cpressure : Fcn  Expr=.8 * u^2
  Friction Drag Calculator : Subsystem
  Product5 : Product
  Sum2 : Sum  Inputs=+++
  Switch : Switch  Criteria=u2 > Threshold  Threshold=1
  Caxial : Outport  VectorParamsAs1DForOutWhenUnconnected=off
  wires:
  Nose Cone Wet Area (m^2)/1 -> Friction Drag Calculator/8(Nose Cone Wet Area (m^2))
  Reference Area (m^2)/1 -> Friction Drag Calculator/10(Reference Area (m^2))
  Reference Radius (m)/1 -> Friction Drag Calculator/9(Reference Radius (m))
  Body Tube Wet Area (m^2)/1 -> Friction Drag Calculator/7(Body Tube Wet Area (m^2))
  sinphi/1 -> Cpressure/1
  Airspeed/1 -> Friction Drag Calculator/5(Airspeed)
  Surface Roughness/1 -> Friction Drag Calculator/4(Surface Roughness)
  Temperature/1 -> Friction Drag Calculator/2(Temperature)
  Mach/1 -> Cbase/1, Cbase1/1, Switch/2, Friction Drag Calculator/11(Mach)
  Density/1 -> Friction Drag Calculator/1(Density)
  Nose Cone Length (m)/1 -> Friction Drag Calculator/3(Nose Cone Length (m))
  Body Tube Length (m)/1 -> Friction Drag Calculator/6(Body Tube Length (m))
  Product5/1 -> Caxial/1
  Friction Drag Calculator/1(CFrictionDrag) -> Sum2/1
  Cbase/1 -> Switch/3
  Cpressure/1 -> Sum2/3
  AoA (rad)/1 -> Axial Drag Multiplier/1(AoA (rads)
  Sum2/1 -> Product5/2
  Axial Drag Multiplier/1(CD Multiplier) -> Product5/1
  Cbase1/1 -> Switch/1
  Switch/1 -> Sum2/2

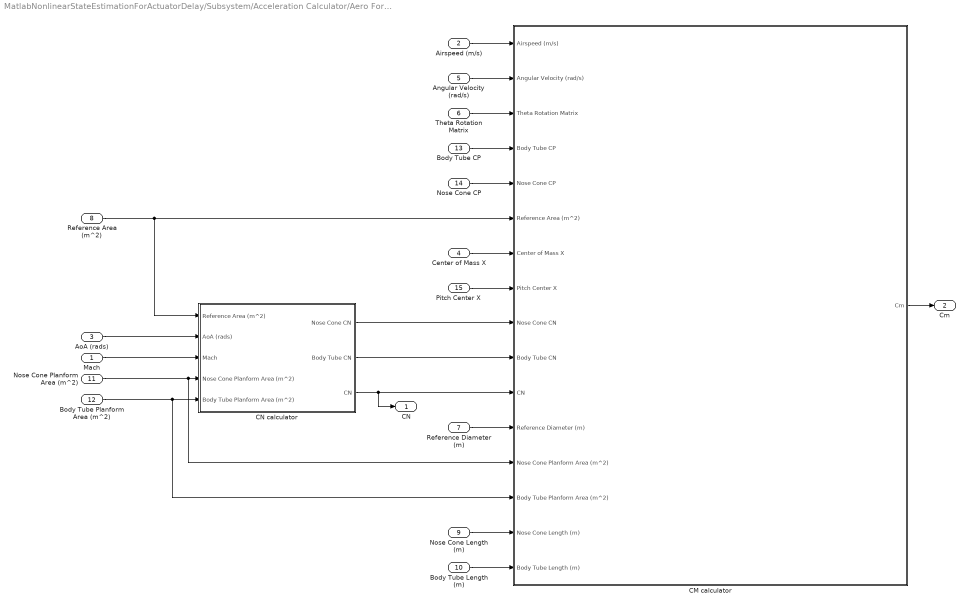
== system MatlabNonlinearStateEstimationForActuatorDelay/Subsystem/Acceleration Calculator/Aero Forces and Moments/CN and Cm calculator ==
  Mach : Inport
  Airspeed (m/s) : Inport  Port=2
  AoA (rads) : Inport  Port=3
  Center of Mass X : Inport  Port=4
  Angular Velocity (rad/s) : Inport  Port=5
  Theta Rotation Matrix : Inport  Port=6
  Reference Diameter (m) : Inport  Port=7
  Reference Area (m^2) : Inport  Port=8
  Nose Cone Length (m) : Inport  Port=9
  Body Tube Length (m) : Inport  Port=10
  Nose Cone Planform Area (m^2) : Inport  Port=11
  Body Tube Planform Area (m^2) : Inport  Port=12
  Body Tube CP : Inport  Port=13
  Nose Cone CP : Inport  Port=14
  Pitch Center X : Inport  Port=15
  CM calculator : Subsystem
  CN calculator : Subsystem
  CN : Outport  VectorParamsAs1DForOutWhenUnconnected=off
  Cm : Outport  Port=2  VectorParamsAs1DForOutWhenUnconnected=off
  wires:
  Body Tube Planform Area (m^2)/1 -> CM calculator/14(Body Tube Planform Area (m^2)), CN calculator/5(Body Tube Planform Area (m^2))
  Pitch Center X/1 -> CM calculator/8(Pitch Center X)
  Nose Cone CP/1 -> CM calculator/5(Nose Cone CP)
  Body Tube CP/1 -> CM calculator/4(Body Tube CP)
  Nose Cone Planform Area (m^2)/1 -> CM calculator/13(Nose Cone Planform Area (m^2)), CN calculator/4(Nose Cone Planform Area (m^2))
  Angular Velocity (rad/s)/1 -> CM calculator/2(Angular Velocity (rad/s))
  Reference Area (m^2)/1 -> CN calculator/1(Reference Area (m^2)), CM calculator/6(Reference Area (m^2))
  AoA (rads)/1 -> CN calculator/2(AoA (rads))
  Mach/1 -> CN calculator/3(Mach)
  Center of Mass X/1 -> CM calculator/7(Center of Mass X)
  CN calculator/3(CN) -> CN/1, CM calculator/11(CN)
  CN calculator/2(Body Tube CN) -> CM calculator/10(Body Tube CN)
  CN calculator/1(Nose Cone CN) -> CM calculator/9(Nose Cone CN)
  Airspeed (m/s)/1 -> CM calculator/1(Airspeed (m/s))
  Theta Rotation Matrix/1 -> CM calculator/3(Theta Rotation Matrix)
  Reference Diameter (m)/1 -> CM calculator/12(Reference Diameter (m))
  Nose Cone Length (m)/1 -> CM calculator/15(Nose Cone Length (m))
  CM calculator/1(Cm) -> Cm/1
  Body Tube Length (m)/1 -> CM calculator/16(Body Tube Length (m))

== system MatlabNonlinearStateEstimationForActuatorDelay/Subsystem/Acceleration Calculator/Aero Forces and Moments/Coefficients to Force ==
  Caxial : Inport
  Cside : Inport  Port=2
  CN : Inport  Port=3
  Theta Rotation : Inport  Port=4
  z : Inport  Port=5
  Aero Forces : Product  Inputs=**  Multiplication=Matrix(*)
  Gain5 : Gain  Gain=-1
  Multiply : Product
  Vector Concatenate3 : Concatenate  NumInputs=3
  Force (N) : Outport  VectorParamsAs1DForOutWhenUnconnected=off
  wires:
  Vector Concatenate3/1 -> Gain5/1
  Gain5/1 -> Multiply/2
  Caxial/1 -> Vector Concatenate3/3
  CN/1 -> Vector Concatenate3/1
  Multiply/1 -> Aero Forces/2
  Aero Forces/1 -> Force (N)/1
  Theta Rotation/1 -> Aero Forces/1
  Cside/1 -> Vector Concatenate3/2
  z/1 -> Multiply/1

== system MatlabNonlinearStateEstimationForActuatorDelay/Subsystem/Acceleration Calculator/Aero Forces and Moments/Coefficients to Moment ==
  z : Inport
  Theta Rotation Matrix : Inport  Port=2
  Cyaw : Inport  Port=3
  Cpitch : Inport  Port=4
  Reference Diameter (m) : Inport  Port=5
  Croll : Inport  Port=6
  Aero Moments : Product  Inputs=**  Multiplication=Matrix(*)
  CNCMxL1 : Product  Inputs=***
  Gain4 : Gain  Gain=-1
  Vector Concatenate4 : Concatenate  NumInputs=3
  Moments (Nm) : Outport  VectorParamsAs1DForOutWhenUnconnected=off
  wires:
  Gain4/1 -> Vector Concatenate4/1
  Vector Concatenate4/1 -> CNCMxL1/2
  Reference Diameter (m)/1 -> CNCMxL1/3
  CNCMxL1/1 -> Aero Moments/2
  Cyaw/1 -> Gain4/1
  Croll/1 -> Vector Concatenate4/3
  z/1 -> CNCMxL1/1
  Theta Rotation Matrix/1 -> Aero Moments/1
  Cpitch/1 -> Vector Concatenate4/2
  Aero Moments/1 -> Moments (Nm)/1

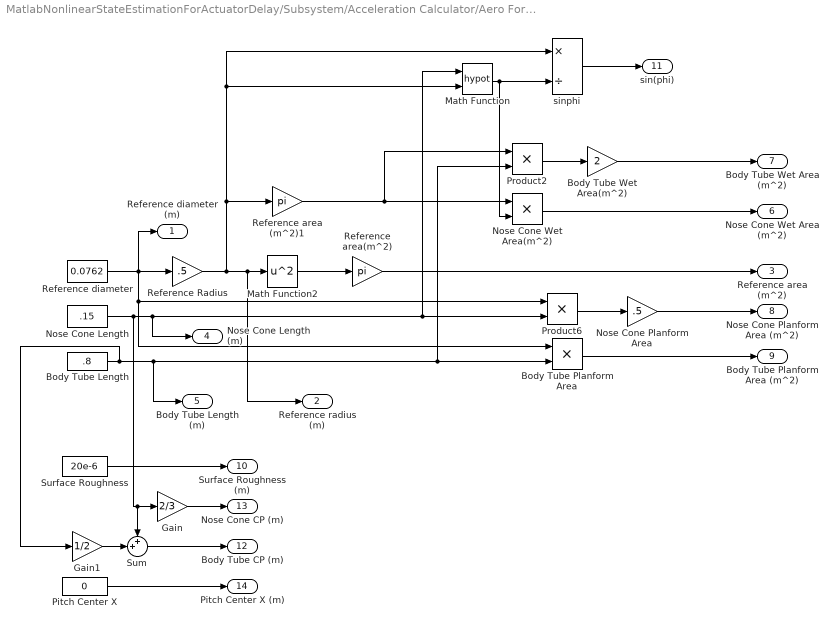
== system MatlabNonlinearStateEstimationForActuatorDelay/Subsystem/Acceleration Calculator/Aero Forces and Moments/Constants ==
  Body Tube Length : Constant  Value=.8
  Body Tube Planform Area : Product
  Body Tube Wet Area(m^2) : Gain  Gain=2
  Gain : Gain  Gain=2/3
  Gain1 : Gain  Gain=1/2
  Math Function : Math  Operator=hypot  SignedPower=on  SaturateOnIntegerOverflow=on
  Math Function2 : Math  Operator=square  SignedPower=on  SaturateOnIntegerOverflow=on
  Nose Cone Length : Constant  Value=.15
  Nose Cone Planform Area : Gain  Gain=.5
  Nose Cone Wet Area(m^2) : Product
  Pitch Center X : Constant  Value=0
  Product2 : Product
  Product6 : Product
  Reference Radius : Gain  Gain=.5
  Reference area (m^2)1 : Gain  Gain=pi
  Reference area(m^2) : Gain  Gain=pi
  Reference diameter : Constant  Value=0.0762
  Sum : Sum  Inputs=++|
  Surface Roughness : Constant  Value=20e-6
  sinphi : Product  Inputs=*/
  Reference diameter (m) : Outport  VectorParamsAs1DForOutWhenUnconnected=off
  Reference radius (m) : Outport  Port=2  VectorParamsAs1DForOutWhenUnconnected=off
  Reference area (m^2) : Outport  Port=3  VectorParamsAs1DForOutWhenUnconnected=off
  Nose Cone Length (m) : Outport  Port=4  VectorParamsAs1DForOutWhenUnconnected=off
  Body Tube Length (m) : Outport  Port=5  VectorParamsAs1DForOutWhenUnconnected=off
  "Nose Cone Wet Area (m^2) " : Outport  Port=6  VectorParamsAs1DForOutWhenUnconnected=off
  Body Tube Wet Area (m^2) : Outport  Port=7  VectorParamsAs1DForOutWhenUnconnected=off
  Nose Cone Planform Area (m^2) : Outport  Port=8  VectorParamsAs1DForOutWhenUnconnected=off
  Body Tube Planform Area (m^2) : Outport  Port=9  VectorParamsAs1DForOutWhenUnconnected=off
  Surface Roughness (m) : Outport  Port=10  VectorParamsAs1DForOutWhenUnconnected=off
  sin(phi) : Outport  Port=11  VectorParamsAs1DForOutWhenUnconnected=off
  Body Tube CP (m) : Outport  Port=12  VectorParamsAs1DForOutWhenUnconnected=off
  Nose Cone CP (m) : Outport  Port=13  VectorParamsAs1DForOutWhenUnconnected=off
  Pitch Center X (m) : Outport  Port=14  VectorParamsAs1DForOutWhenUnconnected=off
  wires:
  Reference diameter/1 -> Reference diameter (m)/1, Body Tube Planform Area/1, Product6/1, Reference Radius/1
  Math Function2/1 -> Reference area(m^2)/1
  Nose Cone Length/1 -> Product6/2, Math Function/1, Nose Cone Length (m)/1, Sum/1, Gain/1
  Product6/1 -> Nose Cone Planform Area/1
  Reference Radius/1 -> Math Function2/1, Reference radius (m)/1, Math Function/2, sinphi/1, Reference area (m^2)1/1
  Reference area (m^2)1/1 -> Product2/1, Nose Cone Wet Area(m^2)/1
  Product2/1 -> Body Tube Wet Area(m^2)/1
  Math Function/1 -> Nose Cone Wet Area(m^2)/2, sinphi/2
  Reference area(m^2)/1 -> Reference area (m^2)/1
  Nose Cone Wet Area(m^2)/1 -> "Nose Cone Wet Area (m^2) "/1
  Body Tube Wet Area(m^2)/1 -> Body Tube Wet Area (m^2)/1
  Body Tube Planform Area/1 -> Body Tube Planform Area (m^2)/1
  Nose Cone Planform Area/1 -> Nose Cone Planform Area (m^2)/1
  Surface Roughness/1 -> Surface Roughness (m)/1
  sinphi/1 -> sin(phi)/1
  Sum/1 -> Body Tube CP (m)/1
  Gain/1 -> Nose Cone CP (m)/1
  Pitch Center X/1 -> Pitch Center X (m)/1
  Gain1/1 -> Sum/2
  Body Tube Length/1 -> Gain1/1, Body Tube Length (m)/1, Body Tube Planform Area/2, Product2/2

== system MatlabNonlinearStateEstimationForActuatorDelay/Subsystem/Acceleration Calculator/Aero Forces and Moments/Theta Rotation ==
  Local Airspeed (m/s) : Inport
  1 : Constant
  Demux : Demux  Outputs=2
  Dot Product : DotProduct  SaturateOnIntegerOverflow=on  OutDataTypeStr=Inherit: Inherit via internal rule
  Gain3 : Gain  Gain=-1
  Ground : Ground
  Theta Rotation : sharedutil/Create 3x3 Matrix  aMode=aMode
      settings: SourceProductBaseCode=AE,PW,MT,UV,VE,VP
  V : Math  Operator=sqrt  SignedPower=on  SaturateOnIntegerOverflow=on
  "cosa, sina" : Product  Inputs=*/
  xy Airspeed : Selector  InputPortWidth=3  IndexOptions=Index vector (dialog)  Indices=[1 2]  OutputSizes=1
  Theta Rotation Matrix : Outport  VectorParamsAs1DForOutWhenUnconnected=off
  wires:
  "cosa, sina"/1 -> Demux/1
  xy Airspeed/1 -> Dot Product/2, Dot Product/1, "cosa, sina"/1
  V/1 -> "cosa, sina"/2
  Demux/1 -> Theta Rotation/5, Theta Rotation/1
  1/1 -> Theta Rotation/9
  Ground/1 -> Theta Rotation/3, Theta Rotation/6, Theta Rotation/7, Theta Rotation/8
  Demux/2 -> Gain3/1, Theta Rotation/4
  Local Airspeed (m/s)/1 -> xy Airspeed/1
  Dot Product/1 -> V/1
  Gain3/1 -> Theta Rotation/2
  Theta Rotation/1 -> Theta Rotation Matrix/1

== system MatlabNonlinearStateEstimationForActuatorDelay/Subsystem/Acceleration Calculator/Subsystem/Subsystem1 ==
  Airspeed : Inport
  Divide : Product  Inputs=*/
  Dot Product : DotProduct  SaturateOnIntegerOverflow=on  OutDataTypeStr=Inherit: Inherit via internal rule
  Sel1 : Selector  IndexMode=Zero-based  InputPortWidth=3  IndexOptions=Index vector (dialog)  Indices=2  OutputSizes=1
  Trigonometric Function : Trigonometry  Operator=acos
  V : Math  Operator=sqrt  SignedPower=on  SaturateOnIntegerOverflow=on
  AoA : Outport  VectorParamsAs1DForOutWhenUnconnected=off
  wires:
  Trigonometric Function/1 -> AoA/1
  Airspeed/1 -> Sel1/1, Dot Product/1, Dot Product/2
  Divide/1 -> Trigonometric Function/1
  Sel1/1 -> Divide/1
  Dot Product/1 -> V/1
  V/1 -> Divide/2

== system MatlabNonlinearStateEstimationForActuatorDelay/Subsystem/Subsystem/Subsystem/Subsystem ==
  p q r1 : Inport
  q0 q1 q2 q1 : Inport  Port=2
  Constant : Constant
  Dot Product : DotProduct  OutDataTypeStr=Inherit: Inherit via internal rule
  High Gain Quaternion Normalization : Gain  SaturateOnIntegerOverflow=on  OutDataTypeStr=Inherit: Same as input  ParamDataTypeStr=Inherit: Same as input
  Mux1 : Mux  Inputs=[3 4 1]
  Mux2 : Mux
  Sum : Sum  Inputs=|+-  InputSameDT=on  SaturateOnIntegerOverflow=on  OutDataTypeStr=Inherit: Same as first input
  q0dot : Fcn  Expr=-0.5 * ( u[5]*u[1]+u[6]*u[2]+u[7]*u[3] ) + u[8]*u[4]
  q1dot : Fcn  Expr=0.5 * ( u[4]*u[1]+u[6]*u[3]-u[7]*u[2] ) + u[8]*u[5]
  q2dot : Fcn  Expr=0.5 * ( u[4]*u[2]+u[7]*u[1]-u[5]*u[3] ) + u[8]*u[6]
  q3dot : Fcn  Expr=0.5 * ( u[4]*u[3]+u[5]*u[2]-u[6]*u[1] ) + u[8]*u[7]
  qdot1 : Outport  InitialOutput=0  VectorParamsAs1DForOutWhenUnconnected=off
  wires:
  Constant/1 -> Sum/1
  Dot Product/1 -> Sum/2
  Mux1/1 -> q2dot/1, q3dot/1, q0dot/1, q1dot/1
  q0 q1 q2 q1/1 -> Dot Product/1, Dot Product/2, Mux1/2
  Sum/1 -> High Gain Quaternion Normalization/1
  Mux2/1 -> qdot1/1
  q0dot/1 -> Mux2/1
  q3dot/1 -> Mux2/4
  q1dot/1 -> Mux2/2
  q2dot/1 -> Mux2/3
  High Gain Quaternion Normalization/1 -> Mux1/3
  p q r1/1 -> Mux1/1

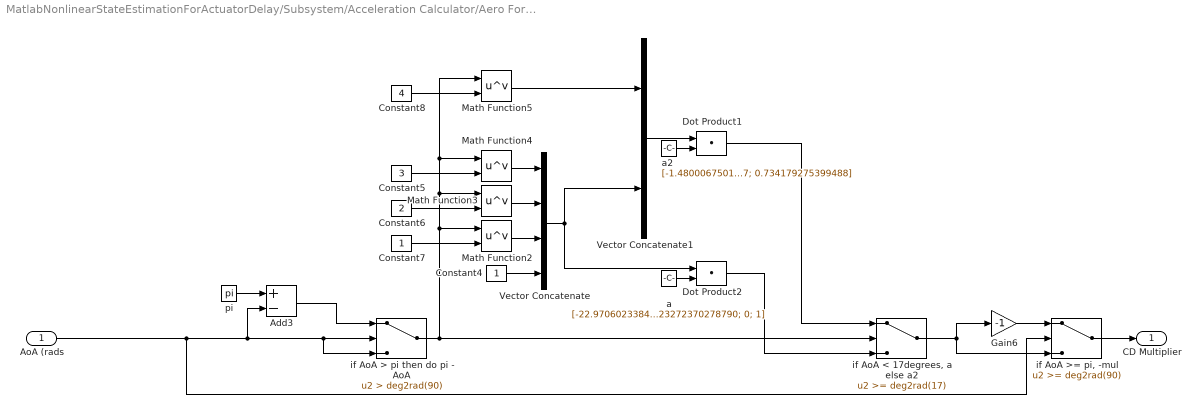
== system MatlabNonlinearStateEstimationForActuatorDelay/Subsystem/Acceleration Calculator/Aero Forces and Moments/Axial Drag Calculator/Axial Drag Multiplier ==
  AoA (rads : Inport
  Add3 : Sum  Inputs=+-
  Constant4 : Constant
  Constant5 : Constant  Value=3
  Constant6 : Constant  Value=2
  Constant7 : Constant
  Constant8 : Constant  Value=4
  Dot Product1 : DotProduct  SaturateOnIntegerOverflow=on  OutDataTypeStr=Inherit: Inherit via internal rule
  Dot Product2 : DotProduct  SaturateOnIntegerOverflow=on  OutDataTypeStr=Inherit: Inherit via internal rule
  Gain6 : Gain  Gain=-1
  Math Function{2..5} (4 alike) : Math  Operator=pow  SignedPower=on  SaturateOnIntegerOverflow=on
  Vector Concatenate : Concatenate  NumInputs=4
  Vector Concatenate1 : Concatenate
  a : Constant  Value=[-22.970602338418825; 10.223272370278790; 0; 1]
  a2 : Constant  Value=[-1.480006750190687; 6.784940235048046; -10.062655893223173; 4.334008218595027; 0.734179275399488]
  "if AoA < 17degrees, a else a2" : Switch  Threshold=deg2rad(17)
  if AoA > pi then do pi - AoA : Switch  Criteria=u2 > Threshold  Threshold=deg2rad(90)
  "if AoA >= pi, -mul" : Switch  Threshold=deg2rad(90)
  pi : Constant  Value=pi
  CD Multiplier : Outport  VectorParamsAs1DForOutWhenUnconnected=off
  wires:
  Constant4/1 -> Vector Concatenate/4
  Constant5/1 -> Math Function4/2
  if AoA > pi then do pi - AoA/1 -> Math Function5/1, Math Function4/1, Math Function3/1, Math Function2/1, "if AoA < 17degrees, a else a2"/2
  Add3/1 -> if AoA > pi then do pi - AoA/1
  Vector Concatenate1/1 -> Dot Product1/1
  AoA (rads/1 -> "if AoA >= pi, -mul"/2, Add3/2, if AoA > pi then do pi - AoA/3, if AoA > pi then do pi - AoA/2
  a/1 -> Dot Product2/2
  "if AoA >= pi, -mul"/1 -> CD Multiplier/1
  Math Function4/1 -> Vector Concatenate/1
  "if AoA < 17degrees, a else a2"/1 -> "if AoA >= pi, -mul"/3, Gain6/1
  Gain6/1 -> "if AoA >= pi, -mul"/1
  pi/1 -> Add3/1
  Constant7/1 -> Math Function2/2
  Vector Concatenate/1 -> Vector Concatenate1/2, Dot Product2/1
  Math Function2/1 -> Vector Concatenate/3
  Constant6/1 -> Math Function3/2
  Dot Product2/1 -> "if AoA < 17degrees, a else a2"/3
  Constant8/1 -> Math Function5/2
  a2/1 -> Dot Product1/2
  Math Function5/1 -> Vector Concatenate1/1
  Math Function3/1 -> Vector Concatenate/2
  Dot Product1/1 -> "if AoA < 17degrees, a else a2"/1
